simulink model "simul4"  (R2023b)
settings: Solver=ode4  StartTime=0.0  StopTime=240  FixedStep=0.004  RelTol=1e-3
InitFcn:
  | start4
StopFcn:
  | stop4
values from neighbouring files (symbols this model uses):
  biais_acc = 0.003    [params4.m]    (also in start4.m)
undefined symbols (not defined in the file or in its folder): a_dlpf, b_dlpf
libraries: simulink x1
settings Model: Creator=xavie  LastModifiedBy=xavie
settings DataIOCC: ReturnWorkspaceOutputs=off

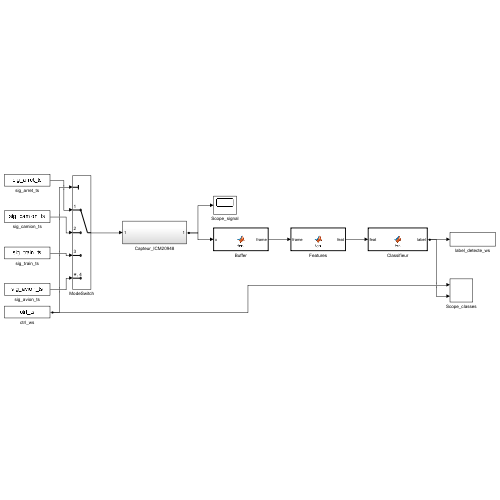
[thumbnail: Simulink's stored preview of the top-level diagram]
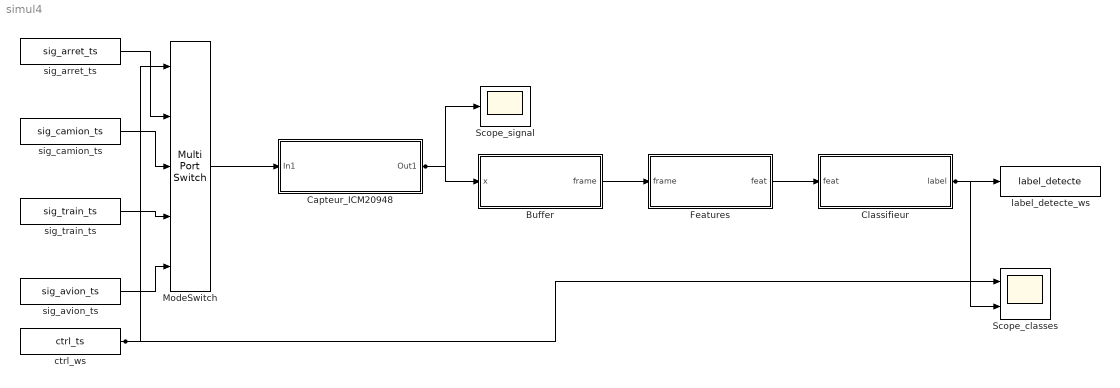
== system simul4 ==
  Buffer : MATLAB Function  TreatAsAtomicUnit=on
  Capteur_ICM20948 : Subsystem
  Classifieur : MATLAB Function  TreatAsAtomicUnit=on
  Features : MATLAB Function  TreatAsAtomicUnit=on
  ModeSwitch : MultiPortSwitch  Inputs=4  SaturateOnIntegerOverflow=off  InputSameDT=off
  Scope_classes : Scope  NumInputPorts=2
  Scope_signal : Scope
  ctrl_ws : FromWorkspace  VariableName=ctrl_ts  SampleTime=0.004  Interpolate=off  OutputAfterFinalValue=Holding final value
  label_detecte_ws : ToWorkspace  VariableName=label_detecte  SampleTime=-1
  sig_arret_ts : FromWorkspace  VariableName=sig_arret_ts  SampleTime=0.004  Interpolate=off  OutputAfterFinalValue=Holding final value
  sig_avion_ts : FromWorkspace  VariableName=sig_avion_ts  SampleTime=0.004  Interpolate=off  OutputAfterFinalValue=Holding final value
  sig_camion_ts : FromWorkspace  VariableName=sig_camion_ts  SampleTime=0.004  Interpolate=off  OutputAfterFinalValue=Holding final value
  sig_train_ts : FromWorkspace  VariableName=sig_train_ts  SampleTime=0.004  Interpolate=off  OutputAfterFinalValue=Holding final value
  wires:
  ctrl_ws/1 -> ModeSwitch/1, Scope_classes/1
  sig_arret_ts/1 -> ModeSwitch/2
  sig_camion_ts/1 -> ModeSwitch/3
  sig_train_ts/1 -> ModeSwitch/4
  sig_avion_ts/1 -> ModeSwitch/5
  ModeSwitch/1 -> Capteur_ICM20948/1(In1)
  Capteur_ICM20948/1(Out1) -> Scope_signal/1, Buffer/1(x)
  Buffer/1(frame) -> Features/1(frame)
  Features/1(feat) -> Classifieur/1(feat)
  Classifieur/1(label) -> label_detecte_ws/1, Scope_classes/2

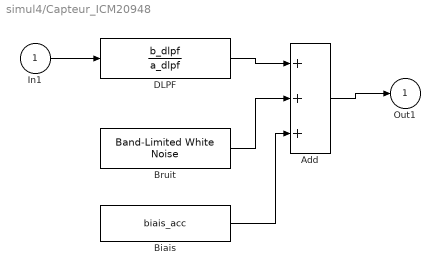
== system simul4/Capteur_ICM20948 ==
  In1 : Inport
  Add : Sum  Inputs=+++
  Biais : Constant  Value=biais_acc
  Bruit : simulink/Sources/Band-Limited White Noise  Cov=7.2e-09  Ts=0.004  seed=4321
  DLPF : DiscreteTransferFcn  Numerator=b_dlpf  Denominator=a_dlpf  SampleTime=0.004
  Out1 : Outport
  wires:
  In1/1 -> DLPF/1
  DLPF/1 -> Add/1
  Bruit/1 -> Add/2
  Biais/1 -> Add/3
  Add/1 -> Out1/1

== matlab function simul4/Buffer ==
  data: x input; frame output
function frame = buffer_fn(x)
%BUFFER_FN  Fenetre glissante 2500 pts, overlap 50%
%  Entree : x      scalaire (1 echantillon a 250 Hz)
%  Sortie : frame  vecteur 2500x1 (nouveau toutes les 1250 entrees, zeros sinon)
%#codegen
N  = int32(2500);
NO = int32(1250);

persistent buf cnt
if isempty(buf)
    buf = zeros(N, 1);
    cnt = int32(0);
end

buf = [buf(2:end); x];
cnt = cnt + int32(1);

% Declaration explicite AVANT le if : Simulink connait la taille de sortie
frame = zeros(N, 1);
if cnt >= NO
    frame = buf;
    cnt   = int32(0);
end
end

== matlab function simul4/Classifieur ==
  data: feat input; label output
function label = classifieur_fn(feat)
%CLASSIFIEUR_FN  Classification k-NN (k=3)
%  Entree : feat   vecteur 1x6 (issu de features_fn)
%  Sortie : label  scalaire 1=Arret 2=Camion 3=Train 4=Avion
%  Le classifieur ne tourne que lorsque feat a change (gain de temps)
coder.extrinsic('predict_wrapper');

persistent last_feat last_label
if isempty(last_feat)
    last_feat  = zeros(1, 6);
    last_label = double(1);
end

% Calcul uniquement si nouvelles features disponibles
if any(feat ~= last_feat)
    last_label = double(0);
    last_label = predict_wrapper(feat);
    last_feat  = feat;
end

label = last_label;
end

== matlab function simul4/Features ==
  data: frame input; feat output
function feat = features_fn(frame)
%FEATURES_FN  Extraction de 6 primitives spectrales sur une fenetre
%  Entree : frame  vecteur 2500x1 (issu de buffer_fn — zeros si pas de nouvelle fenetre)
%  Sortie : feat   vecteur 1x6 [RMS, crete, f_centroid, E_basse, E_milieu, E_haute]
%  La FFT n'est calculee que lorsque frame est non nul (~ 48 fois sur 240s)
%#codegen
fs_loc = 250;
N_loc  = 2500;

persistent last_feat
if isempty(last_feat)
    last_feat = zeros(1, 6);
end

% Calcul uniquement si nouvelle fenetre (frame non nul)
if frame(1) ~= 0 || frame(N_loc) ~= 0
    x = frame;

    rms_val  = sqrt(mean(x.^2));
    crete    = max(abs(x)) / (rms_val + 1e-12);

    X_fft    = abs(fft(x)).^2 / (N_loc * fs_loc);
    X_one    = X_fft(1:N_loc/2+1);
    X_one(2:end-1) = 2 * X_one(2:end-1);
    f_v      = (0:N_loc/2)' * fs_loc / N_loc;
    df_loc   = fs_loc / N_loc;
    E_tot    = sum(X_one) * df_loc + 1e-12;

    f_c      = sum(f_v .* X_one) * df_loc / E_tot;
    E_basse  = sum(X_one(f_v >= 1  & f_v <  5 )) * df_loc / E_tot;
    E_milieu = sum(X_one(f_v >= 5  & f_v < 50 )) * df_loc / E_tot;
    E_haute  = sum(X_one(f_v >= 50 & f_v < 125)) * df_loc / E_tot;

    last_feat = [rms_val, crete, f_c, E_basse, E_milieu, E_haute];
end

feat = last_feat;
end
